simulink model "state_space_all_reduce_uio"  (R2018a)
settings: Solver=FixedStepAuto  StartTime=0.0  StopTime=3  FixedStep=tm  MaxStep=1e-4  RelTol=1e-5  AbsTol=1e-5
InitFcn:
  | SimulinkInit_linea_transmision
values from neighbouring files (symbols this model uses):
  b = 4.91    [SimulinkInit_linea_transmision.m]
  C = 1    [SimulinkInit_linea_transmision.m]
  C1 = 22e-6    (= 2.2e-05)    [SimulinkInit_linea_transmision.m]
  C2 = 22e-6    (= 2.2e-05)    [SimulinkInit_linea_transmision.m]
  C3 = 610e-6    (= 0.00061)    [SimulinkInit_linea_transmision.m]
  Cl = 20000e-6    (= 0.02)    [SimulinkInit_linea_transmision.m]
  Jd = 0.3    [SimulinkInit_linea_transmision.m]
  K = 25    [SimulinkInit_linea_transmision.m]    (also in uio_linear.m = K1+E*H)
  K1 = 9.66    [SimulinkInit_linea_transmision.m]    (also in uio_linear.m = K1')
  K11 = 0.8    [SimulinkInit_linea_transmision.m]
  K1d = 1.15    [SimulinkInit_linea_transmision.m]
  K2 = 6.97    [SimulinkInit_linea_transmision.m]
  K22 = 0.2    [SimulinkInit_linea_transmision.m]
  K2d = 1    [SimulinkInit_linea_transmision.m]
  K3 = 31.8    [SimulinkInit_linea_transmision.m]
  K33 = 0.23    [SimulinkInit_linea_transmision.m]
  K3d = 1    [SimulinkInit_linea_transmision.m]
  K4 = 15.1    [SimulinkInit_linea_transmision.m]
  Kd = 0.02    [SimulinkInit_linea_transmision.m]
  Kdc = 0.02    [SimulinkInit_linea_transmision.m]
  Kf = 1    [SimulinkInit_linea_transmision.m]
  Kh = 1.2    [SimulinkInit_linea_transmision.m]
  Ks = 21.5    [SimulinkInit_linea_transmision.m]
  Ksc = 3    [SimulinkInit_linea_transmision.m]
  Kv = 1    [SimulinkInit_linea_transmision.m]
  L = 5.2    [SimulinkInit_linea_transmision.m]
  L1 = 40e-3    (= 0.04)    [SimulinkInit_linea_transmision.m]
  L2 = 30e-3    (= 0.03)    [SimulinkInit_linea_transmision.m]
  L3 = 5e-3    (= 0.005)    [SimulinkInit_linea_transmision.m]
  L4 = 35e-6    (= 3.5e-05)    [SimulinkInit_linea_transmision.m]
  L5 = 22e-6    (= 2.2e-05)    [SimulinkInit_linea_transmision.m]
  L6 = 10e-6    (= 1e-05)    [SimulinkInit_linea_transmision.m]
  Pd = 0.1    [SimulinkInit_linea_transmision.m]
  R = 10    [SimulinkInit_linea_transmision.m]
  R1 = 0.1    [SimulinkInit_linea_transmision.m]
  R2 = 0.2    [SimulinkInit_linea_transmision.m]
  R3 = 1e-3    (= 0.001)    [SimulinkInit_linea_transmision.m]
  R4 = 0.005    [SimulinkInit_linea_transmision.m]
  R5 = 0.0012    [SimulinkInit_linea_transmision.m]
  R6 = 0.001    [SimulinkInit_linea_transmision.m]
  RL = 10    [SimulinkInit_linea_transmision.m]
  Sbin = 13.8    [SimulinkInit_linea_transmision.m]
  Svin = 2.91    [SimulinkInit_linea_transmision.m]
  T1 = 0.4    [SimulinkInit_linea_transmision.m]
  T2 = 1    [SimulinkInit_linea_transmision.m]
  T3 = 15    [SimulinkInit_linea_transmision.m]
  T4 = 2.5    [SimulinkInit_linea_transmision.m]
  Tao1d = 0.5    [SimulinkInit_linea_transmision.m]
  Tao2d = 0.125    [SimulinkInit_linea_transmision.m]
  Tcd = 0.2    [SimulinkInit_linea_transmision.m]
  Tcr = 0.01    [SimulinkInit_linea_transmision.m]
  Tf = 0.04    [SimulinkInit_linea_transmision.m]
  Tr = 950    [SimulinkInit_linea_transmision.m]
  Tt = 450    [SimulinkInit_linea_transmision.m]
  Ttd = 0.04    [SimulinkInit_linea_transmision.m]
  Tv = 0.05    [SimulinkInit_linea_transmision.m]
  V = 20    [SimulinkInit_linea_transmision.m]
  wref = 70000    [SimulinkInit_linea_transmision.m]
  X_acid = 1.2    [SimulinkInit_linea_transmision.m]
  X_meth = 0.35    [SimulinkInit_linea_transmision.m]
  Z = 3    [SimulinkInit_linea_transmision.m]
undefined symbols (not defined in the file or in its folder): Ad, ataque, Bd, c11, c12, c13, c14, C1o, c21, c22, c23, c24, C2o, c31, c32, c33, c34, C3o, c41, c42, c43, c44, C4o, Cd, F1, F2, F3, F4, H1, H2, H3, H4, K1U, K2U, K3U, K4U, T1s, T2s, T3s, T4s, T5s, tao1, tao2, taod, tm, uio1r, uio2r, uio3r, uio4r
libraries: neural x277, dsparch4 x4, powerlib_meascontrol x4, mpclib x1, simulink x1
(part 4 of 16)

== system state_space_all_reduce_uio/Function Fitting Neural Network2/Layer 2 ==
  "a{1} " : Inport  PortDimensions=30  SampleTime=4e-05
      mask Display: e = 0.06;c1 = [120 230 180]/255;c2 = ([120 230 180]+0)/(256+128);c3 = ([120 230 180]+128)/(256+128);patch([0 1 1 0],[0 0 1 1],c1);patch([0 1 1 1-e 1-e 0+e],[0 0 1 1-e 0+e 0+e],c2);patch([0 0 1 1-e 0+e 0+e],[0 1 1 1-e 1-e 0+e],c3);plot([0 1 1 0 0],[0 0 1 1 0]);
  Delays 1 : Subsystem
      mask Display: e = 0.06;c1 = [120 150 230]/255;c2 = ([120 150 230]+0)/383;c3 = ([120 150 230]+128)/383;patch([0 1 1 0],[0 0 1 1],c1);patch([0 1 1 1-e 1-e 0+e],[0 0 1 1-e 0+e 0+e],c2);patch([0 0 1 1-e 0+e 0+e],[0 1 1 1-e 1-e 0+e],c3);plot([0 1 1 0 0],[0 0 1 1 0]);disp('0');
  "LW{2,1}" : Subsystem
      mask Display: e = 0.06;c1 = [120 150 230]/255;c2 = ([120 150 230]+0)/383;c3 = ([120 150 230]+128)/383;patch([0 1 1 0],[0 0 1 1],c1);patch([0 1 1 1-e 1-e 0+e],[0 0 1 1-e 0+e 0+e],c2);patch([0 0 1 1-e 0+e 0+e],[0 1 1 1-e 1-e 0+e],c3);plot([0 1 1 0 0],[0 0 1 1 0]);disp('W');
  "b{2}" : Constant  Value=[-1.56797212552154352493971600779332220554351806640625;-1.173172027791388405404404693399555981159210205078125;-0.84861883917887592776452265752595849335193634033203125;0.5012025349146498331975863038678653538227081298828125;-0.1471121592091874930030570567396352998912334442138671875;0.18435318847665793651202648106846027076244354248046875;-0.449273547762377212233531054152990691363811492919921875;0.81641684595448271721807032008655369281768798828125;1.20088065217263295636485054274089634418487548828125;1.5110993013098983350772641642834059894084930419921875]
      mask Display: e = 0.06;c1 = [120 150 230]/255;c2 = ([120 150 230]+0)/383;c3 = ([120 150 230]+128)/383;patch([0 1 1 0],[0 0 1 1],c1);patch([0 1 1 1-e 1-e 0+e],[0 0 1 1-e 0+e 0+e],c2);patch([0 0 1 1-e 0+e 0+e],[0 1 1 1-e 1-e 0+e],c3);plot([0 1 1 0 0],[0 0 1 1 0]);disp('b');
  netsum : Sum  Inputs=2  SaturateOnIntegerOverflow=on  InputSameDT=on  OutDataTypeStr=Inherit: Same as first input
      mask Display: e = 0.06;c1 = [120 150 230]/255;c2 = ([120 150 230]+0)/383;c3 = ([120 150 230]+128)/383;patch([0 1 1 0],[0 0 1 1],c1);patch([0 1 1 1-e 1-e 0+e],[0 0 1 1-e 0+e 0+e],c2);patch([0 0 1 1-e 0+e 0+e],[0 1 1 1-e 1-e 0+e],c3);plot([0 1 1 0 0],[0 0 1 1 0]);disp('+');
  tansig : neural/Transfer Functions/tansig
  "a{2}" : Outport  InitialOutput=[0;0;0;0;0;0;0;0;0;0]
      mask Display: e = 0.06;c1 = [120 230 180]/255;c2 = ([120 230 180]+0)/(256+128);c3 = ([120 230 180]+128)/(256+128);patch([0 1 1 0],[0 0 1 1],c1);patch([0 1 1 1-e 1-e 0+e],[0 0 1 1-e 0+e 0+e],c2);patch([0 0 1 1-e 0+e 0+e],[0 1 1 1-e 1-e 0+e],c3);plot([0 1 1 0 0],[0 0 1 1 0]);
  wires:
  "a{1} "/1 -> Delays 1/1("p{2}")
  Delays 1/1("pd{2,1}") -> "LW{2,1}"/1("ad{2,1}")
  "LW{2,1}"/1("lz{2,1}") -> netsum/1
  "b{2}"/1 -> netsum/2
  netsum/1 -> tansig/1
  tansig/1 -> "a{2}"/1

== system state_space_all_reduce_uio/Function Fitting Neural Network2/Layer 3 ==
  "a{2} " : Inport  PortDimensions=10  SampleTime=4e-05
      mask Display: e = 0.06;c1 = [120 230 180]/255;c2 = ([120 230 180]+0)/(256+128);c3 = ([120 230 180]+128)/(256+128);patch([0 1 1 0],[0 0 1 1],c1);patch([0 1 1 1-e 1-e 0+e],[0 0 1 1-e 0+e 0+e],c2);patch([0 0 1 1-e 0+e 0+e],[0 1 1 1-e 1-e 0+e],c3);plot([0 1 1 0 0],[0 0 1 1 0]);
  Delays 1 : Subsystem
      mask Display: e = 0.06;c1 = [120 150 230]/255;c2 = ([120 150 230]+0)/383;c3 = ([120 150 230]+128)/383;patch([0 1 1 0],[0 0 1 1],c1);patch([0 1 1 1-e 1-e 0+e],[0 0 1 1-e 0+e 0+e],c2);patch([0 0 1 1-e 0+e 0+e],[0 1 1 1-e 1-e 0+e],c3);plot([0 1 1 0 0],[0 0 1 1 0]);disp('0');
  "LW{3,2}" : Subsystem
      mask Display: e = 0.06;c1 = [120 150 230]/255;c2 = ([120 150 230]+0)/383;c3 = ([120 150 230]+128)/383;patch([0 1 1 0],[0 0 1 1],c1);patch([0 1 1 1-e 1-e 0+e],[0 0 1 1-e 0+e 0+e],c2);patch([0 0 1 1-e 0+e 0+e],[0 1 1 1-e 1-e 0+e],c3);plot([0 1 1 0 0],[0 0 1 1 0]);disp('W');
  "b{3}" : Constant  Value=[1.8223455275545192844077746485709212720394134521484375;1.43060627453565825106807096744887530803680419921875;-1.0023903103419706805965461171581409871578216552734375;-0.6759509023179954834148475129040889441967010498046875;-0.1975460742379759049303089568638824857771396636962890625;0.179200247261637468643158399572712369263172149658203125;-0.54043828705023588820921531805652193725109100341796875;0.9844996358065831731920525271561928093433380126953125;-1.3852814991285520296315780797158367931842803955078125;-1.7150106273510032917073431235621683299541473388671875]
      mask Display: e = 0.06;c1 = [120 150 230]/255;c2 = ([120 150 230]+0)/383;c3 = ([120 150 230]+128)/383;patch([0 1 1 0],[0 0 1 1],c1);patch([0 1 1 1-e 1-e 0+e],[0 0 1 1-e 0+e 0+e],c2);patch([0 0 1 1-e 0+e 0+e],[0 1 1 1-e 1-e 0+e],c3);plot([0 1 1 0 0],[0 0 1 1 0]);disp('b');
  netsum : Sum  Inputs=2  SaturateOnIntegerOverflow=on  InputSameDT=on  OutDataTypeStr=Inherit: Same as first input
      mask Display: e = 0.06;c1 = [120 150 230]/255;c2 = ([120 150 230]+0)/383;c3 = ([120 150 230]+128)/383;patch([0 1 1 0],[0 0 1 1],c1);patch([0 1 1 1-e 1-e 0+e],[0 0 1 1-e 0+e 0+e],c2);patch([0 0 1 1-e 0+e 0+e],[0 1 1 1-e 1-e 0+e],c3);plot([0 1 1 0 0],[0 0 1 1 0]);disp('+');
  tansig : neural/Transfer Functions/tansig
  "a{3}" : Outport  InitialOutput=[0;0;0;0;0;0;0;0;0;0]
      mask Display: e = 0.06;c1 = [120 230 180]/255;c2 = ([120 230 180]+0)/(256+128);c3 = ([120 230 180]+128)/(256+128);patch([0 1 1 0],[0 0 1 1],c1);patch([0 1 1 1-e 1-e 0+e],[0 0 1 1-e 0+e 0+e],c2);patch([0 0 1 1-e 0+e 0+e],[0 1 1 1-e 1-e 0+e],c3);plot([0 1 1 0 0],[0 0 1 1 0]);
  wires:
  "a{2} "/1 -> Delays 1/1("p{3}")
  Delays 1/1("pd{3,2}") -> "LW{3,2}"/1("ad{3,2}")
  "LW{3,2}"/1("lz{3,2}") -> netsum/1
  "b{3}"/1 -> netsum/2
  netsum/1 -> tansig/1
  tansig/1 -> "a{3}"/1

== system state_space_all_reduce_uio/Function Fitting Neural Network2/Layer 4 ==
  "a{3} " : Inport  PortDimensions=10  SampleTime=4e-05
      mask Display: e = 0.06;c1 = [120 230 180]/255;c2 = ([120 230 180]+0)/(256+128);c3 = ([120 230 180]+128)/(256+128);patch([0 1 1 0],[0 0 1 1],c1);patch([0 1 1 1-e 1-e 0+e],[0 0 1 1-e 0+e 0+e],c2);patch([0 0 1 1-e 0+e 0+e],[0 1 1 1-e 1-e 0+e],c3);plot([0 1 1 0 0],[0 0 1 1 0]);
  Delays 1 : Subsystem
      mask Display: e = 0.06;c1 = [120 150 230]/255;c2 = ([120 150 230]+0)/383;c3 = ([120 150 230]+128)/383;patch([0 1 1 0],[0 0 1 1],c1);patch([0 1 1 1-e 1-e 0+e],[0 0 1 1-e 0+e 0+e],c2);patch([0 0 1 1-e 0+e 0+e],[0 1 1 1-e 1-e 0+e],c3);plot([0 1 1 0 0],[0 0 1 1 0]);disp('0');
  "LW{4,3}" : Subsystem
      mask Display: e = 0.06;c1 = [120 150 230]/255;c2 = ([120 150 230]+0)/383;c3 = ([120 150 230]+128)/383;patch([0 1 1 0],[0 0 1 1],c1);patch([0 1 1 1-e 1-e 0+e],[0 0 1 1-e 0+e 0+e],c2);patch([0 0 1 1-e 0+e 0+e],[0 1 1 1-e 1-e 0+e],c3);plot([0 1 1 0 0],[0 0 1 1 0]);disp('W');
  "b{4}" : Constant  Value=-0.8863411196048975870809272237238474190235137939453125
      mask Display: e = 0.06;c1 = [120 150 230]/255;c2 = ([120 150 230]+0)/383;c3 = ([120 150 230]+128)/383;patch([0 1 1 0],[0 0 1 1],c1);patch([0 1 1 1-e 1-e 0+e],[0 0 1 1-e 0+e 0+e],c2);patch([0 0 1 1-e 0+e 0+e],[0 1 1 1-e 1-e 0+e],c3);plot([0 1 1 0 0],[0 0 1 1 0]);disp('b');
  netsum : Sum  Inputs=2  SaturateOnIntegerOverflow=on  InputSameDT=on  OutDataTypeStr=Inherit: Same as first input
      mask Display: e = 0.06;c1 = [120 150 230]/255;c2 = ([120 150 230]+0)/383;c3 = ([120 150 230]+128)/383;patch([0 1 1 0],[0 0 1 1],c1);patch([0 1 1 1-e 1-e 0+e],[0 0 1 1-e 0+e 0+e],c2);patch([0 0 1 1-e 0+e 0+e],[0 1 1 1-e 1-e 0+e],c3);plot([0 1 1 0 0],[0 0 1 1 0]);disp('+');
  purelin : neural/Transfer Functions/purelin
  "a{4}" : Outport  InitialOutput=0
      mask Display: e = 0.06;c1 = [120 230 180]/255;c2 = ([120 230 180]+0)/(256+128);c3 = ([120 230 180]+128)/(256+128);patch([0 1 1 0],[0 0 1 1],c1);patch([0 1 1 1-e 1-e 0+e],[0 0 1 1-e 0+e 0+e],c2);patch([0 0 1 1-e 0+e 0+e],[0 1 1 1-e 1-e 0+e],c3);plot([0 1 1 0 0],[0 0 1 1 0]);
  wires:
  "a{3} "/1 -> Delays 1/1("p{4}")
  Delays 1/1("pd{4,3}") -> "LW{4,3}"/1("ad{4,3}")
  "LW{4,3}"/1("lz{4,3}") -> netsum/1
  "b{4}"/1 -> netsum/2
  netsum/1 -> purelin/1
  purelin/1 -> "a{4}"/1

== system state_space_all_reduce_uio/Function Fitting Neural Network2/Process Input 1 ==
  x : Inport  PortDimensions=44  SampleTime=4e-05
      mask Display: e = 0.06;c1 = [120 230 180]/255;c2 = ([120 230 180]+0)/(256+128);c3 = ([120 230 180]+128)/(256+128);patch([0 1 1 0],[0 0 1 1],c1);patch([0 1 1 1-e 1-e 0+e],[0 0 1 1-e 0+e 0+e],c2);patch([0 0 1 1-e 0+e 0+e],[0 1 1 1-e 1-e 0+e],c3);plot([0 1 1 0 0],[0 0 1 1 0]);
  mapminmax : neural/Processing Functions/mapminmax  xmin=[-51.1014550674109955252788495272;-51.1014550674109955252788495272;-51.1014550674109955252788495272;-51.1014550674109955252788495272;-51.1014550674109955252788495272;-51.1014550674109955252788495272;-51.1014550674109955252788495272;-51.1014550674109955252788495272;-51.1014550674109955252788495272;-51.1014550674109955252788495272;-51.1014550674109955252788495272;-959.19791052449454582529142499;-43.3111724721229691681401163805;-43.3111724721229691681401163805;-43.3111724721229691681401163805;-43.3111724721229691681401163805;-959.19791052449454582529142499;-43.3111724721229691681401163805;-43.3111724721229691681401163805;-43.3111724721229691681401163805;-43.3111724721229691681401163805;-43.3111724721229691681401163805;-23694.5539757817568897735327482;-51.1014550674109955252788495272;-51.1014550674109955252788495272;-51.1014550674109955252788495272;-51.1014550674109955252788495272;-23694.5539757817568897735327482;-51.1014550674109955252788495272;-51.1014550674109955252788495272;-51.1014550674109955252788495272;-51.1014550674109955252788495272;-51.1014550674109955252788495272;-2483.05485238305982420570217073;-1372.04941365416402732080314308;-1372.04941365416402732080314308;-1372.04941365416402732080314308;-1372.04941365416402732080314308;-2483.05485238305982420570217073;-1372.04941365416402732080314308;-1372.04941365416402732080314308;-1372.04941365416402732080314308;-1372.04941365416402732080314308;-1372.04941365416402732080314308]  xmax=[336.625532870159929643705254421;336.625532870159929643705254421;336.625532870159929643705254421;336.625532870159929643705254421;336.625532870159929643705254421;336.625532870159929643705254421;336.625532870159929643705254421;336.625532870159929643705254421;336.625532870159929643705254421;336.625532870159929643705254421;336.625532870159929643705254421;2272.84306749095321720233187079;124.082374617438773611866054125;124.082374617438773611866054125;124.082374617438773611866054125;124.082374617438773611866054125;40200.0234698361382470466196537;124.082374617438773611866054125;124.082374617438773611866054125;124.082374617438773611866054125;124.082374617438773611866054125;124.082374617438773611866054125;934.78555592286670616886112839;336.625532870159929643705254421;336.625532870159929643705254421;336.625532870159929643705254421;336.625532870159929643705254421;96480.0622239970398368313908577;336.625532870159929643705254421;336.625532870159929643705254421;336.625532870159929643705254421;336.625532870159929643705254421;336.625532870159929643705254421;2489.92267124135287303943186998;1344.02443744788956792035605758;1344.02443744788956792035605758;1344.02443744788956792035605758;1344.02443744788956792035605758;2489.92267124135287303943186998;1344.02443744788956792035605758;1344.02443744788956792035605758;1344.02443744788956792035605758;1344.02443744788956792035605758;1344.02443744788956792035605758]  ymin=-1  ymax=1
  p : Outport  PortDimensions=44  SampleTime=4e-05
      mask Display: e = 0.06;c1 = [120 230 180]/255;c2 = ([120 230 180]+0)/(256+128);c3 = ([120 230 180]+128)/(256+128);patch([0 1 1 0],[0 0 1 1],c1);patch([0 1 1 1-e 1-e 0+e],[0 0 1 1-e 0+e 0+e],c2);patch([0 0 1 1-e 0+e 0+e],[0 1 1 1-e 1-e 0+e],c3);plot([0 1 1 0 0],[0 0 1 1 0]);
  wires:
  x/1 -> mapminmax/1
  mapminmax/1 -> p/1

== system state_space_all_reduce_uio/Function Fitting Neural Network2/Process Output 1 ==
  a : Inport  PortDimensions=1  SampleTime=4e-05
      mask Display: e = 0.06;c1 = [120 230 180]/255;c2 = ([120 230 180]+0)/(256+128);c3 = ([120 230 180]+128)/(256+128);patch([0 1 1 0],[0 0 1 1],c1);patch([0 1 1 1-e 1-e 0+e],[0 0 1 1-e 0+e 0+e],c2);patch([0 0 1 1-e 0+e 0+e],[0 1 1 1-e 1-e 0+e],c3);plot([0 1 1 0 0],[0 0 1 1 0]);
  mapminmax_reverse : neural/Processing Functions/mapminmax_reverse  xmin=-51.1014550674109955252788495272  xmax=336.625532870159929643705254421  ymin=-1  ymax=1
  y : Outport  PortDimensions=1  SampleTime=4e-05
      mask Display: e = 0.06;c1 = [120 230 180]/255;c2 = ([120 230 180]+0)/(256+128);c3 = ([120 230 180]+128)/(256+128);patch([0 1 1 0],[0 0 1 1],c1);patch([0 1 1 1-e 1-e 0+e],[0 0 1 1-e 0+e 0+e],c2);patch([0 0 1 1-e 0+e 0+e],[0 1 1 1-e 1-e 0+e],c3);plot([0 1 1 0 0],[0 0 1 1 0]);
  wires:
  a/1 -> mapminmax_reverse/1
  mapminmax_reverse/1 -> y/1

== system state_space_all_reduce_uio/Function Fitting Neural Network3/Layer 1 ==
  "p{1}" : Inport  PortDimensions=44  SampleTime=4e-05
      mask Display: e = 0.06;c1 = [120 230 180]/255;c2 = ([120 230 180]+0)/(256+128);c3 = ([120 230 180]+128)/(256+128);patch([0 1 1 0],[0 0 1 1],c1);patch([0 1 1 1-e 1-e 0+e],[0 0 1 1-e 0+e 0+e],c2);patch([0 0 1 1-e 0+e 0+e],[0 1 1 1-e 1-e 0+e],c3);plot([0 1 1 0 0],[0 0 1 1 0]);
  Delays 1 : Subsystem
      mask Display: e = 0.06;c1 = [120 150 230]/255;c2 = ([120 150 230]+0)/383;c3 = ([120 150 230]+128)/383;patch([0 1 1 0],[0 0 1 1],c1);patch([0 1 1 1-e 1-e 0+e],[0 0 1 1-e 0+e 0+e],c2);patch([0 0 1 1-e 0+e 0+e],[0 1 1 1-e 1-e 0+e],c3);plot([0 1 1 0 0],[0 0 1 1 0]);disp('0');
  "IW{1,1}" : Subsystem
      mask Display: e = 0.06;c1 = [120 150 230]/255;c2 = ([120 150 230]+0)/383;c3 = ([120 150 230]+128)/383;patch([0 1 1 0],[0 0 1 1],c1);patch([0 1 1 1-e 1-e 0+e],[0 0 1 1-e 0+e 0+e],c2);patch([0 0 1 1-e 0+e 0+e],[0 1 1 1-e 1-e 0+e],c3);plot([0 1 1 0 0],[0 0 1 1 0]);disp('W');
  "b{1}" : Constant  Value=[-1.704763521919084201527994082425720989704132080078125;1.4935062934862097794308510856353677809238433837890625;-1.3106157065531676142455808076192624866962432861328125;1.2925856850658075103410737938247621059417724609375;-1.03521023518372690119804246933199465274810791015625;0.79322318311022588233072383445687592029571533203125;-0.98335447842776135818354532602825202047824859619140625;-0.730751430115515798746628206572495400905609130859375;0.6560359659321999270531478032353334128856658935546875;-0.606651771340228851414622113225050270557403564453125;-0.5627410083162776022192019809153862297534942626953125;-0.37770066738225327451772272979724220931529998779296875;0.225263217285463557271185663921642117202281951904296875;0.5116322028066797589218595021520741283893585205078125;0.064624850777566800186235695946379564702510833740234375;0.0277818133398159104741065306143354973755776882171630859375;0.284772308019548725521730148102506063878536224365234375;-0.1474291488661283455741113357362337410449981689453125;-0.448600974398027874112671042894362471997737884521484375;-0.465666201522838496540401820311672054231166839599609375;0.715989746856539710506694973446428775787353515625;-0.71553436706509432330136633026995696127414703369140625;-0.76467697218161756467225131927989423274993896484375;-0.721010267435951757164502851082943379878997802734375;-0.7416306194383743832787558858399279415607452392578125;-1.2266529590046262310210067880689166486263275146484375;1.2213025690121173116864383700885809957981109619140625;1.328009388144533620135234741610474884510040283203125;1.16012996826200076583290865528397262096405029296875;-1.45824071317467751640606365981511771678924560546875]
      mask Display: e = 0.06;c1 = [120 150 230]/255;c2 = ([120 150 230]+0)/383;c3 = ([120 150 230]+128)/383;patch([0 1 1 0],[0 0 1 1],c1);patch([0 1 1 1-e 1-e 0+e],[0 0 1 1-e 0+e 0+e],c2);patch([0 0 1 1-e 0+e 0+e],[0 1 1 1-e 1-e 0+e],c3);plot([0 1 1 0 0],[0 0 1 1 0]);disp('b');
  netsum : Sum  Inputs=2  SaturateOnIntegerOverflow=on  InputSameDT=on  OutDataTypeStr=Inherit: Same as first input
      mask Display: e = 0.06;c1 = [120 150 230]/255;c2 = ([120 150 230]+0)/383;c3 = ([120 150 230]+128)/383;patch([0 1 1 0],[0 0 1 1],c1);patch([0 1 1 1-e 1-e 0+e],[0 0 1 1-e 0+e 0+e],c2);patch([0 0 1 1-e 0+e 0+e],[0 1 1 1-e 1-e 0+e],c3);plot([0 1 1 0 0],[0 0 1 1 0]);disp('+');
  tansig : neural/Transfer Functions/tansig
  "a{1}" : Outport  InitialOutput=[0;0;0;0;0;0;0;0;0;0;0;0;0;0;0;0;0;0;0;0;0;0;0;0;0;0;0;0;0;0]
      mask Display: e = 0.06;c1 = [120 230 180]/255;c2 = ([120 230 180]+0)/(256+128);c3 = ([120 230 180]+128)/(256+128);patch([0 1 1 0],[0 0 1 1],c1);patch([0 1 1 1-e 1-e 0+e],[0 0 1 1-e 0+e 0+e],c2);patch([0 0 1 1-e 0+e 0+e],[0 1 1 1-e 1-e 0+e],c3);plot([0 1 1 0 0],[0 0 1 1 0]);
  wires:
  "p{1}"/1 -> Delays 1/1("p{1}")
  Delays 1/1("pd{1,1}") -> "IW{1,1}"/1("pd{1,1}")
  "IW{1,1}"/1("iz{1,1}") -> netsum/1
  "b{1}"/1 -> netsum/2
  netsum/1 -> tansig/1
  tansig/1 -> "a{1}"/1

== system state_space_all_reduce_uio/Function Fitting Neural Network3/Layer 2 ==
  "a{1} " : Inport  PortDimensions=30  SampleTime=4e-05
      mask Display: e = 0.06;c1 = [120 230 180]/255;c2 = ([120 230 180]+0)/(256+128);c3 = ([120 230 180]+128)/(256+128);patch([0 1 1 0],[0 0 1 1],c1);patch([0 1 1 1-e 1-e 0+e],[0 0 1 1-e 0+e 0+e],c2);patch([0 0 1 1-e 0+e 0+e],[0 1 1 1-e 1-e 0+e],c3);plot([0 1 1 0 0],[0 0 1 1 0]);
  Delays 1 : Subsystem
      mask Display: e = 0.06;c1 = [120 150 230]/255;c2 = ([120 150 230]+0)/383;c3 = ([120 150 230]+128)/383;patch([0 1 1 0],[0 0 1 1],c1);patch([0 1 1 1-e 1-e 0+e],[0 0 1 1-e 0+e 0+e],c2);patch([0 0 1 1-e 0+e 0+e],[0 1 1 1-e 1-e 0+e],c3);plot([0 1 1 0 0],[0 0 1 1 0]);disp('0');
  "LW{2,1}" : Subsystem
      mask Display: e = 0.06;c1 = [120 150 230]/255;c2 = ([120 150 230]+0)/383;c3 = ([120 150 230]+128)/383;patch([0 1 1 0],[0 0 1 1],c1);patch([0 1 1 1-e 1-e 0+e],[0 0 1 1-e 0+e 0+e],c2);patch([0 0 1 1-e 0+e 0+e],[0 1 1 1-e 1-e 0+e],c3);plot([0 1 1 0 0],[0 0 1 1 0]);disp('W');
  "b{2}" : Constant  Value=[1.73453608952175120094807425630278885364532470703125;0.96907661744661732772243567524128593504428863525390625;-0.99021766109755737783615359148825518786907196044921875;0.46812702702532160703441377336275763809680938720703125;0.12300528029318967548899621533564641140401363372802734375;0.03195273129913174525729147035235655494034290313720703125;0.54767140464927177578857708795112557709217071533203125;0.8426375749309331641967446557828225195407867431640625;-0.995458450042752129860446075326763093471527099609375;1.5851687558301594815901580659556202590465545654296875]
      mask Display: e = 0.06;c1 = [120 150 230]/255;c2 = ([120 150 230]+0)/383;c3 = ([120 150 230]+128)/383;patch([0 1 1 0],[0 0 1 1],c1);patch([0 1 1 1-e 1-e 0+e],[0 0 1 1-e 0+e 0+e],c2);patch([0 0 1 1-e 0+e 0+e],[0 1 1 1-e 1-e 0+e],c3);plot([0 1 1 0 0],[0 0 1 1 0]);disp('b');
  netsum : Sum  Inputs=2  SaturateOnIntegerOverflow=on  InputSameDT=on  OutDataTypeStr=Inherit: Same as first input
      mask Display: e = 0.06;c1 = [120 150 230]/255;c2 = ([120 150 230]+0)/383;c3 = ([120 150 230]+128)/383;patch([0 1 1 0],[0 0 1 1],c1);patch([0 1 1 1-e 1-e 0+e],[0 0 1 1-e 0+e 0+e],c2);patch([0 0 1 1-e 0+e 0+e],[0 1 1 1-e 1-e 0+e],c3);plot([0 1 1 0 0],[0 0 1 1 0]);disp('+');
  tansig : neural/Transfer Functions/tansig
  "a{2}" : Outport  InitialOutput=[0;0;0;0;0;0;0;0;0;0]
      mask Display: e = 0.06;c1 = [120 230 180]/255;c2 = ([120 230 180]+0)/(256+128);c3 = ([120 230 180]+128)/(256+128);patch([0 1 1 0],[0 0 1 1],c1);patch([0 1 1 1-e 1-e 0+e],[0 0 1 1-e 0+e 0+e],c2);patch([0 0 1 1-e 0+e 0+e],[0 1 1 1-e 1-e 0+e],c3);plot([0 1 1 0 0],[0 0 1 1 0]);
  wires:
  "a{1} "/1 -> Delays 1/1("p{2}")
  Delays 1/1("pd{2,1}") -> "LW{2,1}"/1("ad{2,1}")
  "LW{2,1}"/1("lz{2,1}") -> netsum/1
  "b{2}"/1 -> netsum/2
  netsum/1 -> tansig/1
  tansig/1 -> "a{2}"/1

== system state_space_all_reduce_uio/Function Fitting Neural Network3/Layer 3 ==
  "a{2} " : Inport  PortDimensions=10  SampleTime=4e-05
      mask Display: e = 0.06;c1 = [120 230 180]/255;c2 = ([120 230 180]+0)/(256+128);c3 = ([120 230 180]+128)/(256+128);patch([0 1 1 0],[0 0 1 1],c1);patch([0 1 1 1-e 1-e 0+e],[0 0 1 1-e 0+e 0+e],c2);patch([0 0 1 1-e 0+e 0+e],[0 1 1 1-e 1-e 0+e],c3);plot([0 1 1 0 0],[0 0 1 1 0]);
  Delays 1 : Subsystem
      mask Display: e = 0.06;c1 = [120 150 230]/255;c2 = ([120 150 230]+0)/383;c3 = ([120 150 230]+128)/383;patch([0 1 1 0],[0 0 1 1],c1);patch([0 1 1 1-e 1-e 0+e],[0 0 1 1-e 0+e 0+e],c2);patch([0 0 1 1-e 0+e 0+e],[0 1 1 1-e 1-e 0+e],c3);plot([0 1 1 0 0],[0 0 1 1 0]);disp('0');
  "LW{3,2}" : Subsystem
      mask Display: e = 0.06;c1 = [120 150 230]/255;c2 = ([120 150 230]+0)/383;c3 = ([120 150 230]+128)/383;patch([0 1 1 0],[0 0 1 1],c1);patch([0 1 1 1-e 1-e 0+e],[0 0 1 1-e 0+e 0+e],c2);patch([0 0 1 1-e 0+e 0+e],[0 1 1 1-e 1-e 0+e],c3);plot([0 1 1 0 0],[0 0 1 1 0]);disp('W');
  "b{3}" : Constant  Value=[-1.603808031376757536889954280923120677471160888671875;1.40202706886736638836055135470815002918243408203125;1.0326256678853507064985706165316514670848846435546875;0.754755996564343778487682357081212103366851806640625;-0.2273936146095133781219743696055957116186618804931640625;0.26644156526305007304245009436272084712982177734375;-0.46750230759845035066746277152560651302337646484375;0.977164184821628367672019521705806255340576171875;-1.39302311135195910907214056351222097873687744140625;-1.95169677096117855086276904330588877201080322265625]
      mask Display: e = 0.06;c1 = [120 150 230]/255;c2 = ([120 150 230]+0)/383;c3 = ([120 150 230]+128)/383;patch([0 1 1 0],[0 0 1 1],c1);patch([0 1 1 1-e 1-e 0+e],[0 0 1 1-e 0+e 0+e],c2);patch([0 0 1 1-e 0+e 0+e],[0 1 1 1-e 1-e 0+e],c3);plot([0 1 1 0 0],[0 0 1 1 0]);disp('b');
  netsum : Sum  Inputs=2  SaturateOnIntegerOverflow=on  InputSameDT=on  OutDataTypeStr=Inherit: Same as first input
      mask Display: e = 0.06;c1 = [120 150 230]/255;c2 = ([120 150 230]+0)/383;c3 = ([120 150 230]+128)/383;patch([0 1 1 0],[0 0 1 1],c1);patch([0 1 1 1-e 1-e 0+e],[0 0 1 1-e 0+e 0+e],c2);patch([0 0 1 1-e 0+e 0+e],[0 1 1 1-e 1-e 0+e],c3);plot([0 1 1 0 0],[0 0 1 1 0]);disp('+');
  tansig : neural/Transfer Functions/tansig
  "a{3}" : Outport  InitialOutput=[0;0;0;0;0;0;0;0;0;0]
      mask Display: e = 0.06;c1 = [120 230 180]/255;c2 = ([120 230 180]+0)/(256+128);c3 = ([120 230 180]+128)/(256+128);patch([0 1 1 0],[0 0 1 1],c1);patch([0 1 1 1-e 1-e 0+e],[0 0 1 1-e 0+e 0+e],c2);patch([0 0 1 1-e 0+e 0+e],[0 1 1 1-e 1-e 0+e],c3);plot([0 1 1 0 0],[0 0 1 1 0]);
  wires:
  "a{2} "/1 -> Delays 1/1("p{3}")
  Delays 1/1("pd{3,2}") -> "LW{3,2}"/1("ad{3,2}")
  "LW{3,2}"/1("lz{3,2}") -> netsum/1
  "b{3}"/1 -> netsum/2
  netsum/1 -> tansig/1
  tansig/1 -> "a{3}"/1

== system state_space_all_reduce_uio/Function Fitting Neural Network3/Layer 4 ==
  "a{3} " : Inport  PortDimensions=10  SampleTime=4e-05
      mask Display: e = 0.06;c1 = [120 230 180]/255;c2 = ([120 230 180]+0)/(256+128);c3 = ([120 230 180]+128)/(256+128);patch([0 1 1 0],[0 0 1 1],c1);patch([0 1 1 1-e 1-e 0+e],[0 0 1 1-e 0+e 0+e],c2);patch([0 0 1 1-e 0+e 0+e],[0 1 1 1-e 1-e 0+e],c3);plot([0 1 1 0 0],[0 0 1 1 0]);
  Delays 1 : Subsystem
      mask Display: e = 0.06;c1 = [120 150 230]/255;c2 = ([120 150 230]+0)/383;c3 = ([120 150 230]+128)/383;patch([0 1 1 0],[0 0 1 1],c1);patch([0 1 1 1-e 1-e 0+e],[0 0 1 1-e 0+e 0+e],c2);patch([0 0 1 1-e 0+e 0+e],[0 1 1 1-e 1-e 0+e],c3);plot([0 1 1 0 0],[0 0 1 1 0]);disp('0');
  "LW{4,3}" : Subsystem
      mask Display: e = 0.06;c1 = [120 150 230]/255;c2 = ([120 150 230]+0)/383;c3 = ([120 150 230]+128)/383;patch([0 1 1 0],[0 0 1 1],c1);patch([0 1 1 1-e 1-e 0+e],[0 0 1 1-e 0+e 0+e],c2);patch([0 0 1 1-e 0+e 0+e],[0 1 1 1-e 1-e 0+e],c3);plot([0 1 1 0 0],[0 0 1 1 0]);disp('W');
  "b{4}" : Constant  Value=-0.7425748194040957539385772179230116307735443115234375
      mask Display: e = 0.06;c1 = [120 150 230]/255;c2 = ([120 150 230]+0)/383;c3 = ([120 150 230]+128)/383;patch([0 1 1 0],[0 0 1 1],c1);patch([0 1 1 1-e 1-e 0+e],[0 0 1 1-e 0+e 0+e],c2);patch([0 0 1 1-e 0+e 0+e],[0 1 1 1-e 1-e 0+e],c3);plot([0 1 1 0 0],[0 0 1 1 0]);disp('b');
  netsum : Sum  Inputs=2  SaturateOnIntegerOverflow=on  InputSameDT=on  OutDataTypeStr=Inherit: Same as first input
      mask Display: e = 0.06;c1 = [120 150 230]/255;c2 = ([120 150 230]+0)/383;c3 = ([120 150 230]+128)/383;patch([0 1 1 0],[0 0 1 1],c1);patch([0 1 1 1-e 1-e 0+e],[0 0 1 1-e 0+e 0+e],c2);patch([0 0 1 1-e 0+e 0+e],[0 1 1 1-e 1-e 0+e],c3);plot([0 1 1 0 0],[0 0 1 1 0]);disp('+');
  purelin : neural/Transfer Functions/purelin
  "a{4}" : Outport  InitialOutput=0
      mask Display: e = 0.06;c1 = [120 230 180]/255;c2 = ([120 230 180]+0)/(256+128);c3 = ([120 230 180]+128)/(256+128);patch([0 1 1 0],[0 0 1 1],c1);patch([0 1 1 1-e 1-e 0+e],[0 0 1 1-e 0+e 0+e],c2);patch([0 0 1 1-e 0+e 0+e],[0 1 1 1-e 1-e 0+e],c3);plot([0 1 1 0 0],[0 0 1 1 0]);
  wires:
  "a{3} "/1 -> Delays 1/1("p{4}")
  Delays 1/1("pd{4,3}") -> "LW{4,3}"/1("ad{4,3}")
  "LW{4,3}"/1("lz{4,3}") -> netsum/1
  "b{4}"/1 -> netsum/2
  netsum/1 -> purelin/1
  purelin/1 -> "a{4}"/1

== system state_space_all_reduce_uio/Function Fitting Neural Network3/Process Input 1 ==
  x : Inport  PortDimensions=44  SampleTime=4e-05
      mask Display: e = 0.06;c1 = [120 230 180]/255;c2 = ([120 230 180]+0)/(256+128);c3 = ([120 230 180]+128)/(256+128);patch([0 1 1 0],[0 0 1 1],c1);patch([0 1 1 1-e 1-e 0+e],[0 0 1 1-e 0+e 0+e],c2);patch([0 0 1 1-e 0+e 0+e],[0 1 1 1-e 1-e 0+e],c3);plot([0 1 1 0 0],[0 0 1 1 0]);
  mapminmax : neural/Processing Functions/mapminmax  xmin=[-1372.04941365416402732080314308;-1372.04941365416402732080314308;-1372.04941365416402732080314308;-1372.04941365416402732080314308;-1372.04941365416402732080314308;-1372.04941365416402732080314308;-1372.04941365416402732080314308;-1372.04941365416402732080314308;-1372.04941365416402732080314308;-1372.04941365416402732080314308;-1372.04941365416402732080314308;-959.19791052449454582529142499;-43.3111724721229691681401163805;-43.3111724721229691681401163805;-43.3111724721229691681401163805;-43.3111724721229691681401163805;-959.19791052449454582529142499;-43.3111724721229691681401163805;-43.3111724721229691681401163805;-43.3111724721229691681401163805;-43.3111724721229691681401163805;-43.3111724721229691681401163805;-23694.5539757817568897735327482;-51.1014550674109955252788495272;-51.1014550674109955252788495272;-51.1014550674109955252788495272;-51.1014550674109955252788495272;-23694.5539757817568897735327482;-51.1014550674109955252788495272;-51.1014550674109955252788495272;-51.1014550674109955252788495272;-51.1014550674109955252788495272;-51.1014550674109955252788495272;-2483.05485238305982420570217073;-1372.04941365416402732080314308;-1372.04941365416402732080314308;-1372.04941365416402732080314308;-1372.04941365416402732080314308;-2483.05485238305982420570217073;-1372.04941365416402732080314308;-1372.04941365416402732080314308;-1372.04941365416402732080314308;-1372.04941365416402732080314308;-1372.04941365416402732080314308]  xmax=[1344.02443744788956792035605758;1344.02443744788956792035605758;1344.02443744788956792035605758;1344.02443744788956792035605758;1344.02443744788956792035605758;1344.02443744788956792035605758;1344.02443744788956792035605758;1344.02443744788956792035605758;1344.02443744788956792035605758;1344.02443744788956792035605758;1344.02443744788956792035605758;2272.84306749095321720233187079;124.082374617438773611866054125;124.082374617438773611866054125;124.082374617438773611866054125;124.082374617438773611866054125;40200.0234698361382470466196537;124.082374617438773611866054125;124.082374617438773611866054125;124.082374617438773611866054125;124.082374617438773611866054125;124.082374617438773611866054125;934.78555592286670616886112839;336.625532870159929643705254421;336.625532870159929643705254421;336.625532870159929643705254421;336.625532870159929643705254421;96480.0622239970398368313908577;336.625532870159929643705254421;336.625532870159929643705254421;336.625532870159929643705254421;336.625532870159929643705254421;336.625532870159929643705254421;2489.92267124135287303943186998;1344.02443744788956792035605758;1344.02443744788956792035605758;1344.02443744788956792035605758;1344.02443744788956792035605758;2489.92267124135287303943186998;1344.02443744788956792035605758;1344.02443744788956792035605758;1344.02443744788956792035605758;1344.02443744788956792035605758;1344.02443744788956792035605758]  ymin=-1  ymax=1
  p : Outport  PortDimensions=44  SampleTime=4e-05
      mask Display: e = 0.06;c1 = [120 230 180]/255;c2 = ([120 230 180]+0)/(256+128);c3 = ([120 230 180]+128)/(256+128);patch([0 1 1 0],[0 0 1 1],c1);patch([0 1 1 1-e 1-e 0+e],[0 0 1 1-e 0+e 0+e],c2);patch([0 0 1 1-e 0+e 0+e],[0 1 1 1-e 1-e 0+e],c3);plot([0 1 1 0 0],[0 0 1 1 0]);
  wires:
  x/1 -> mapminmax/1
  mapminmax/1 -> p/1

== system state_space_all_reduce_uio/Function Fitting Neural Network3/Process Output 1 ==
  a : Inport  PortDimensions=1  SampleTime=4e-05
      mask Display: e = 0.06;c1 = [120 230 180]/255;c2 = ([120 230 180]+0)/(256+128);c3 = ([120 230 180]+128)/(256+128);patch([0 1 1 0],[0 0 1 1],c1);patch([0 1 1 1-e 1-e 0+e],[0 0 1 1-e 0+e 0+e],c2);patch([0 0 1 1-e 0+e 0+e],[0 1 1 1-e 1-e 0+e],c3);plot([0 1 1 0 0],[0 0 1 1 0]);
  mapminmax_reverse : neural/Processing Functions/mapminmax_reverse  xmin=-1372.04941365416402732080314308  xmax=1344.02443744788956792035605758  ymin=-1  ymax=1
  y : Outport  PortDimensions=1  SampleTime=4e-05
      mask Display: e = 0.06;c1 = [120 230 180]/255;c2 = ([120 230 180]+0)/(256+128);c3 = ([120 230 180]+128)/(256+128);patch([0 1 1 0],[0 0 1 1],c1);patch([0 1 1 1-e 1-e 0+e],[0 0 1 1-e 0+e 0+e],c2);patch([0 0 1 1-e 0+e 0+e],[0 1 1 1-e 1-e 0+e],c3);plot([0 1 1 0 0],[0 0 1 1 0]);
  wires:
  a/1 -> mapminmax_reverse/1
  mapminmax_reverse/1 -> y/1

== system state_space_all_reduce_uio/Function Fitting Neural Network4/Layer 1 ==
  "p{1}" : Inport  PortDimensions=44  SampleTime=4e-05
      mask Display: e = 0.06;c1 = [120 230 180]/255;c2 = ([120 230 180]+0)/(256+128);c3 = ([120 230 180]+128)/(256+128);patch([0 1 1 0],[0 0 1 1],c1);patch([0 1 1 1-e 1-e 0+e],[0 0 1 1-e 0+e 0+e],c2);patch([0 0 1 1-e 0+e 0+e],[0 1 1 1-e 1-e 0+e],c3);plot([0 1 1 0 0],[0 0 1 1 0]);
  Delays 1 : Subsystem
      mask Display: e = 0.06;c1 = [120 150 230]/255;c2 = ([120 150 230]+0)/383;c3 = ([120 150 230]+128)/383;patch([0 1 1 0],[0 0 1 1],c1);patch([0 1 1 1-e 1-e 0+e],[0 0 1 1-e 0+e 0+e],c2);patch([0 0 1 1-e 0+e 0+e],[0 1 1 1-e 1-e 0+e],c3);plot([0 1 1 0 0],[0 0 1 1 0]);disp('0');
  "IW{1,1}" : Subsystem
      mask Display: e = 0.06;c1 = [120 150 230]/255;c2 = ([120 150 230]+0)/383;c3 = ([120 150 230]+128)/383;patch([0 1 1 0],[0 0 1 1],c1);patch([0 1 1 1-e 1-e 0+e],[0 0 1 1-e 0+e 0+e],c2);patch([0 0 1 1-e 0+e 0+e],[0 1 1 1-e 1-e 0+e],c3);plot([0 1 1 0 0],[0 0 1 1 0]);disp('W');
  "b{1}" : Constant  Value=[1.0374409035086957775462224162765778601169586181640625;-1.707514409991484516382342917495407164096832275390625;-0.70444312940589004501390490986523218452930450439453125;2.12517551426123230129405783372931182384490966796875;-0.87278446469294568288432856206782162189483642578125;1.0638441235973987719631850268342532217502593994140625;-0.52309173161666400186931014104629866778850555419921875;-0.86003587405303727475569530724897049367427825927734375;0.442077018396996146432087471112026832997798919677734375;-0.245349869863336345066073818088625557720661163330078125;0.276031222455307145846603589234291575849056243896484375;-0.8349534119849140179070445810793898999691009521484375;0.0103625387742495335408055012749173329211771488189697265625;0.28181158260352834332707061548717319965362548828125;-0.7084692692417731141318881782353855669498443603515625;0.42470579079327563931656186468899250030517578125;0.08184375275959841766759694792199297808110713958740234375;-0.385317630502477637133296184401842765510082244873046875;-0.8065938937915058115635247304453514516353607177734375;0.79626062283174448008793433473329059779644012451171875;1.0448912937651464449828608849202282726764678955078125;-0.433575220525991233966323079584981314837932586669921875;-0.78357793365093264537080131049151532351970672607421875;1.3837732276238716710992093794629909098148345947265625;1.871700143481612510498734991415403783321380615234375;-1.419290850209196985787230005371384322643280029296875;-1.2072392041524044881128929773694835603237152099609375;0.8328927652172166684607645947835408151149749755859375;1.9384602649459752310434623723267577588558197021484375;-1.7475711827877133952569010943989269435405731201171875]
      mask Display: e = 0.06;c1 = [120 150 230]/255;c2 = ([120 150 230]+0)/383;c3 = ([120 150 230]+128)/383;patch([0 1 1 0],[0 0 1 1],c1);patch([0 1 1 1-e 1-e 0+e],[0 0 1 1-e 0+e 0+e],c2);patch([0 0 1 1-e 0+e 0+e],[0 1 1 1-e 1-e 0+e],c3);plot([0 1 1 0 0],[0 0 1 1 0]);disp('b');
  netsum : Sum  Inputs=2  SaturateOnIntegerOverflow=on  InputSameDT=on  OutDataTypeStr=Inherit: Same as first input
      mask Display: e = 0.06;c1 = [120 150 230]/255;c2 = ([120 150 230]+0)/383;c3 = ([120 150 230]+128)/383;patch([0 1 1 0],[0 0 1 1],c1);patch([0 1 1 1-e 1-e 0+e],[0 0 1 1-e 0+e 0+e],c2);patch([0 0 1 1-e 0+e 0+e],[0 1 1 1-e 1-e 0+e],c3);plot([0 1 1 0 0],[0 0 1 1 0]);disp('+');
  tansig : neural/Transfer Functions/tansig
  "a{1}" : Outport  InitialOutput=[0;0;0;0;0;0;0;0;0;0;0;0;0;0;0;0;0;0;0;0;0;0;0;0;0;0;0;0;0;0]
      mask Display: e = 0.06;c1 = [120 230 180]/255;c2 = ([120 230 180]+0)/(256+128);c3 = ([120 230 180]+128)/(256+128);patch([0 1 1 0],[0 0 1 1],c1);patch([0 1 1 1-e 1-e 0+e],[0 0 1 1-e 0+e 0+e],c2);patch([0 0 1 1-e 0+e 0+e],[0 1 1 1-e 1-e 0+e],c3);plot([0 1 1 0 0],[0 0 1 1 0]);
  wires:
  "p{1}"/1 -> Delays 1/1("p{1}")
  Delays 1/1("pd{1,1}") -> "IW{1,1}"/1("pd{1,1}")
  "IW{1,1}"/1("iz{1,1}") -> netsum/1
  "b{1}"/1 -> netsum/2
  netsum/1 -> tansig/1
  tansig/1 -> "a{1}"/1

== system state_space_all_reduce_uio/Function Fitting Neural Network4/Layer 2 ==
  "a{1} " : Inport  PortDimensions=30  SampleTime=4e-05
      mask Display: e = 0.06;c1 = [120 230 180]/255;c2 = ([120 230 180]+0)/(256+128);c3 = ([120 230 180]+128)/(256+128);patch([0 1 1 0],[0 0 1 1],c1);patch([0 1 1 1-e 1-e 0+e],[0 0 1 1-e 0+e 0+e],c2);patch([0 0 1 1-e 0+e 0+e],[0 1 1 1-e 1-e 0+e],c3);plot([0 1 1 0 0],[0 0 1 1 0]);
  Delays 1 : Subsystem
      mask Display: e = 0.06;c1 = [120 150 230]/255;c2 = ([120 150 230]+0)/383;c3 = ([120 150 230]+128)/383;patch([0 1 1 0],[0 0 1 1],c1);patch([0 1 1 1-e 1-e 0+e],[0 0 1 1-e 0+e 0+e],c2);patch([0 0 1 1-e 0+e 0+e],[0 1 1 1-e 1-e 0+e],c3);plot([0 1 1 0 0],[0 0 1 1 0]);disp('0');
  "LW{2,1}" : Subsystem
      mask Display: e = 0.06;c1 = [120 150 230]/255;c2 = ([120 150 230]+0)/383;c3 = ([120 150 230]+128)/383;patch([0 1 1 0],[0 0 1 1],c1);patch([0 1 1 1-e 1-e 0+e],[0 0 1 1-e 0+e 0+e],c2);patch([0 0 1 1-e 0+e 0+e],[0 1 1 1-e 1-e 0+e],c3);plot([0 1 1 0 0],[0 0 1 1 0]);disp('W');
  "b{2}" : Constant  Value=[1.3298337406165712248906629611155949532985687255859375;-0.60403765953027865887037251013680361211299896240234375;0.7540564819898627479943797879968769848346710205078125;0.1677828591221107445985438744173734448850154876708984375;0.83934372728013972864147262953338213264942169189453125;-0.2817999444816801091207025820040144026279449462890625;-1.0432027939087500367776328857871703803539276123046875;-0.413595722473691862486333548076800070703029632568359375;0.934438725760213362292461170000024139881134033203125;1.018458753690340667930058771162293851375579833984375]
      mask Display: e = 0.06;c1 = [120 150 230]/255;c2 = ([120 150 230]+0)/383;c3 = ([120 150 230]+128)/383;patch([0 1 1 0],[0 0 1 1],c1);patch([0 1 1 1-e 1-e 0+e],[0 0 1 1-e 0+e 0+e],c2);patch([0 0 1 1-e 0+e 0+e],[0 1 1 1-e 1-e 0+e],c3);plot([0 1 1 0 0],[0 0 1 1 0]);disp('b');
  netsum : Sum  Inputs=2  SaturateOnIntegerOverflow=on  InputSameDT=on  OutDataTypeStr=Inherit: Same as first input
      mask Display: e = 0.06;c1 = [120 150 230]/255;c2 = ([120 150 230]+0)/383;c3 = ([120 150 230]+128)/383;patch([0 1 1 0],[0 0 1 1],c1);patch([0 1 1 1-e 1-e 0+e],[0 0 1 1-e 0+e 0+e],c2);patch([0 0 1 1-e 0+e 0+e],[0 1 1 1-e 1-e 0+e],c3);plot([0 1 1 0 0],[0 0 1 1 0]);disp('+');
  tansig : neural/Transfer Functions/tansig
  "a{2}" : Outport  InitialOutput=[0;0;0;0;0;0;0;0;0;0]
      mask Display: e = 0.06;c1 = [120 230 180]/255;c2 = ([120 230 180]+0)/(256+128);c3 = ([120 230 180]+128)/(256+128);patch([0 1 1 0],[0 0 1 1],c1);patch([0 1 1 1-e 1-e 0+e],[0 0 1 1-e 0+e 0+e],c2);patch([0 0 1 1-e 0+e 0+e],[0 1 1 1-e 1-e 0+e],c3);plot([0 1 1 0 0],[0 0 1 1 0]);
  wires:
  "a{1} "/1 -> Delays 1/1("p{2}")
  Delays 1/1("pd{2,1}") -> "LW{2,1}"/1("ad{2,1}")
  "LW{2,1}"/1("lz{2,1}") -> netsum/1
  "b{2}"/1 -> netsum/2
  netsum/1 -> tansig/1
  tansig/1 -> "a{2}"/1

== system state_space_all_reduce_uio/Function Fitting Neural Network4/Layer 3 ==
  "a{2} " : Inport  PortDimensions=10  SampleTime=4e-05
      mask Display: e = 0.06;c1 = [120 230 180]/255;c2 = ([120 230 180]+0)/(256+128);c3 = ([120 230 180]+128)/(256+128);patch([0 1 1 0],[0 0 1 1],c1);patch([0 1 1 1-e 1-e 0+e],[0 0 1 1-e 0+e 0+e],c2);patch([0 0 1 1-e 0+e 0+e],[0 1 1 1-e 1-e 0+e],c3);plot([0 1 1 0 0],[0 0 1 1 0]);
  Delays 1 : Subsystem
      mask Display: e = 0.06;c1 = [120 150 230]/255;c2 = ([120 150 230]+0)/383;c3 = ([120 150 230]+128)/383;patch([0 1 1 0],[0 0 1 1],c1);patch([0 1 1 1-e 1-e 0+e],[0 0 1 1-e 0+e 0+e],c2);patch([0 0 1 1-e 0+e 0+e],[0 1 1 1-e 1-e 0+e],c3);plot([0 1 1 0 0],[0 0 1 1 0]);disp('0');
  "LW{3,2}" : Subsystem
      mask Display: e = 0.06;c1 = [120 150 230]/255;c2 = ([120 150 230]+0)/383;c3 = ([120 150 230]+128)/383;patch([0 1 1 0],[0 0 1 1],c1);patch([0 1 1 1-e 1-e 0+e],[0 0 1 1-e 0+e 0+e],c2);patch([0 0 1 1-e 0+e 0+e],[0 1 1 1-e 1-e 0+e],c3);plot([0 1 1 0 0],[0 0 1 1 0]);disp('W');
  "b{3}" : Constant  Value=[-2.031066127256160758207670369301922619342803955078125;-1.4858359983643680823917065936257131397724151611328125;0.1424579958208725682933248890549293719232082366943359375;0.07641397275605743555360049867886118590831756591796875;0.016317364905767121896484894705281476490199565887451171875;-0.860343202250315020052084946655668318271636962890625;1.3324165557267313442224576647276990115642547607421875;-2.739092480878635882390881306491792201995849609375;-1.642884070686016162454734512721188366413116455078125;-0.63510890992286495038143812053021974861621856689453125]
      mask Display: e = 0.06;c1 = [120 150 230]/255;c2 = ([120 150 230]+0)/383;c3 = ([120 150 230]+128)/383;patch([0 1 1 0],[0 0 1 1],c1);patch([0 1 1 1-e 1-e 0+e],[0 0 1 1-e 0+e 0+e],c2);patch([0 0 1 1-e 0+e 0+e],[0 1 1 1-e 1-e 0+e],c3);plot([0 1 1 0 0],[0 0 1 1 0]);disp('b');
  netsum : Sum  Inputs=2  SaturateOnIntegerOverflow=on  InputSameDT=on  OutDataTypeStr=Inherit: Same as first input
      mask Display: e = 0.06;c1 = [120 150 230]/255;c2 = ([120 150 230]+0)/383;c3 = ([120 150 230]+128)/383;patch([0 1 1 0],[0 0 1 1],c1);patch([0 1 1 1-e 1-e 0+e],[0 0 1 1-e 0+e 0+e],c2);patch([0 0 1 1-e 0+e 0+e],[0 1 1 1-e 1-e 0+e],c3);plot([0 1 1 0 0],[0 0 1 1 0]);disp('+');
  tansig : neural/Transfer Functions/tansig
  "a{3}" : Outport  InitialOutput=[0;0;0;0;0;0;0;0;0;0]
      mask Display: e = 0.06;c1 = [120 230 180]/255;c2 = ([120 230 180]+0)/(256+128);c3 = ([120 230 180]+128)/(256+128);patch([0 1 1 0],[0 0 1 1],c1);patch([0 1 1 1-e 1-e 0+e],[0 0 1 1-e 0+e 0+e],c2);patch([0 0 1 1-e 0+e 0+e],[0 1 1 1-e 1-e 0+e],c3);plot([0 1 1 0 0],[0 0 1 1 0]);
  wires:
  "a{2} "/1 -> Delays 1/1("p{3}")
  Delays 1/1("pd{3,2}") -> "LW{3,2}"/1("ad{3,2}")
  "LW{3,2}"/1("lz{3,2}") -> netsum/1
  "b{3}"/1 -> netsum/2
  netsum/1 -> tansig/1
  tansig/1 -> "a{3}"/1

== system state_space_all_reduce_uio/Function Fitting Neural Network4/Layer 4 ==
  "a{3} " : Inport  PortDimensions=10  SampleTime=4e-05
      mask Display: e = 0.06;c1 = [120 230 180]/255;c2 = ([120 230 180]+0)/(256+128);c3 = ([120 230 180]+128)/(256+128);patch([0 1 1 0],[0 0 1 1],c1);patch([0 1 1 1-e 1-e 0+e],[0 0 1 1-e 0+e 0+e],c2);patch([0 0 1 1-e 0+e 0+e],[0 1 1 1-e 1-e 0+e],c3);plot([0 1 1 0 0],[0 0 1 1 0]);
  Delays 1 : Subsystem
      mask Display: e = 0.06;c1 = [120 150 230]/255;c2 = ([120 150 230]+0)/383;c3 = ([120 150 230]+128)/383;patch([0 1 1 0],[0 0 1 1],c1);patch([0 1 1 1-e 1-e 0+e],[0 0 1 1-e 0+e 0+e],c2);patch([0 0 1 1-e 0+e 0+e],[0 1 1 1-e 1-e 0+e],c3);plot([0 1 1 0 0],[0 0 1 1 0]);disp('0');
  "LW{4,3}" : Subsystem
      mask Display: e = 0.06;c1 = [120 150 230]/255;c2 = ([120 150 230]+0)/383;c3 = ([120 150 230]+128)/383;patch([0 1 1 0],[0 0 1 1],c1);patch([0 1 1 1-e 1-e 0+e],[0 0 1 1-e 0+e 0+e],c2);patch([0 0 1 1-e 0+e 0+e],[0 1 1 1-e 1-e 0+e],c3);plot([0 1 1 0 0],[0 0 1 1 0]);disp('W');
  "b{4}" : Constant  Value=0.627556427457597099106578752980567514896392822265625
      mask Display: e = 0.06;c1 = [120 150 230]/255;c2 = ([120 150 230]+0)/383;c3 = ([120 150 230]+128)/383;patch([0 1 1 0],[0 0 1 1],c1);patch([0 1 1 1-e 1-e 0+e],[0 0 1 1-e 0+e 0+e],c2);patch([0 0 1 1-e 0+e 0+e],[0 1 1 1-e 1-e 0+e],c3);plot([0 1 1 0 0],[0 0 1 1 0]);disp('b');
  netsum : Sum  Inputs=2  SaturateOnIntegerOverflow=on  InputSameDT=on  OutDataTypeStr=Inherit: Same as first input
      mask Display: e = 0.06;c1 = [120 150 230]/255;c2 = ([120 150 230]+0)/383;c3 = ([120 150 230]+128)/383;patch([0 1 1 0],[0 0 1 1],c1);patch([0 1 1 1-e 1-e 0+e],[0 0 1 1-e 0+e 0+e],c2);patch([0 0 1 1-e 0+e 0+e],[0 1 1 1-e 1-e 0+e],c3);plot([0 1 1 0 0],[0 0 1 1 0]);disp('+');
  purelin : neural/Transfer Functions/purelin
  "a{4}" : Outport  InitialOutput=0
      mask Display: e = 0.06;c1 = [120 230 180]/255;c2 = ([120 230 180]+0)/(256+128);c3 = ([120 230 180]+128)/(256+128);patch([0 1 1 0],[0 0 1 1],c1);patch([0 1 1 1-e 1-e 0+e],[0 0 1 1-e 0+e 0+e],c2);patch([0 0 1 1-e 0+e 0+e],[0 1 1 1-e 1-e 0+e],c3);plot([0 1 1 0 0],[0 0 1 1 0]);
  wires:
  "a{3} "/1 -> Delays 1/1("p{4}")
  Delays 1/1("pd{4,3}") -> "LW{4,3}"/1("ad{4,3}")
  "LW{4,3}"/1("lz{4,3}") -> netsum/1
  "b{4}"/1 -> netsum/2
  netsum/1 -> purelin/1
  purelin/1 -> "a{4}"/1

== system state_space_all_reduce_uio/Function Fitting Neural Network4/Process Input 1 ==
  x : Inport  PortDimensions=44  SampleTime=4e-05
      mask Display: e = 0.06;c1 = [120 230 180]/255;c2 = ([120 230 180]+0)/(256+128);c3 = ([120 230 180]+128)/(256+128);patch([0 1 1 0],[0 0 1 1],c1);patch([0 1 1 1-e 1-e 0+e],[0 0 1 1-e 0+e 0+e],c2);patch([0 0 1 1-e 0+e 0+e],[0 1 1 1-e 1-e 0+e],c3);plot([0 1 1 0 0],[0 0 1 1 0]);
  mapminmax : neural/Processing Functions/mapminmax  xmin=[-188.063913059203656530371517874;-188.063913059203656530371517874;-188.063913059203656530371517874;-188.063913059203656530371517874;-188.063913059203656530371517874;-188.063913059203656530371517874;-188.063913059203656530371517874;-188.063913059203656530371517874;-188.063913059203656530371517874;-188.063913059203656530371517874;-188.063913059203656530371517874;-959.19791052449454582529142499;-43.3111724721229691681401163805;-43.3111724721229691681401163805;-43.3111724721229691681401163805;-43.3111724721229691681401163805;-959.19791052449454582529142499;-43.3111724721229691681401163805;-43.3111724721229691681401163805;-43.3111724721229691681401163805;-43.3111724721229691681401163805;-43.3111724721229691681401163805;-23694.5539757817568897735327482;-51.1014550674109955252788495272;-51.1014550674109955252788495272;-51.1014550674109955252788495272;-51.1014550674109955252788495272;-23694.5539757817568897735327482;-51.1014550674109955252788495272;-51.1014550674109955252788495272;-51.1014550674109955252788495272;-51.1014550674109955252788495272;-51.1014550674109955252788495272;-2483.05485238305982420570217073;-1372.04941365416402732080314308;-1372.04941365416402732080314308;-1372.04941365416402732080314308;-1372.04941365416402732080314308;-2483.05485238305982420570217073;-1372.04941365416402732080314308;-1372.04941365416402732080314308;-1372.04941365416402732080314308;-1372.04941365416402732080314308;-1372.04941365416402732080314308]  xmax=[193.189082036407143050382728688;193.189082036407143050382728688;193.189082036407143050382728688;193.189082036407143050382728688;193.189082036407143050382728688;193.189082036407143050382728688;193.189082036407143050382728688;193.189082036407143050382728688;193.189082036407143050382728688;193.189082036407143050382728688;193.189082036407143050382728688;2272.84306749095321720233187079;124.082374617438773611866054125;124.082374617438773611866054125;124.082374617438773611866054125;124.082374617438773611866054125;40200.0234698361382470466196537;124.082374617438773611866054125;124.082374617438773611866054125;124.082374617438773611866054125;124.082374617438773611866054125;124.082374617438773611866054125;934.78555592286670616886112839;336.625532870159929643705254421;336.625532870159929643705254421;336.625532870159929643705254421;336.625532870159929643705254421;96480.0622239970398368313908577;336.625532870159929643705254421;336.625532870159929643705254421;336.625532870159929643705254421;336.625532870159929643705254421;336.625532870159929643705254421;2489.92267124135287303943186998;1344.02443744788956792035605758;1344.02443744788956792035605758;1344.02443744788956792035605758;1344.02443744788956792035605758;2489.92267124135287303943186998;1344.02443744788956792035605758;1344.02443744788956792035605758;1344.02443744788956792035605758;1344.02443744788956792035605758;1344.02443744788956792035605758]  ymin=-1  ymax=1
  p : Outport  PortDimensions=44  SampleTime=4e-05
      mask Display: e = 0.06;c1 = [120 230 180]/255;c2 = ([120 230 180]+0)/(256+128);c3 = ([120 230 180]+128)/(256+128);patch([0 1 1 0],[0 0 1 1],c1);patch([0 1 1 1-e 1-e 0+e],[0 0 1 1-e 0+e 0+e],c2);patch([0 0 1 1-e 0+e 0+e],[0 1 1 1-e 1-e 0+e],c3);plot([0 1 1 0 0],[0 0 1 1 0]);
  wires:
  x/1 -> mapminmax/1
  mapminmax/1 -> p/1
